simulink model "untitled"  (R2021a)
settings: Solver=FixedStepAuto  StartTime=0.0  StopTime=20  FixedStep=0.1  RelTol=1e-3
undefined symbols (not defined in the file): sigbuilder_block
settings Model: Creator=se108102  LastModifiedBy=se108102

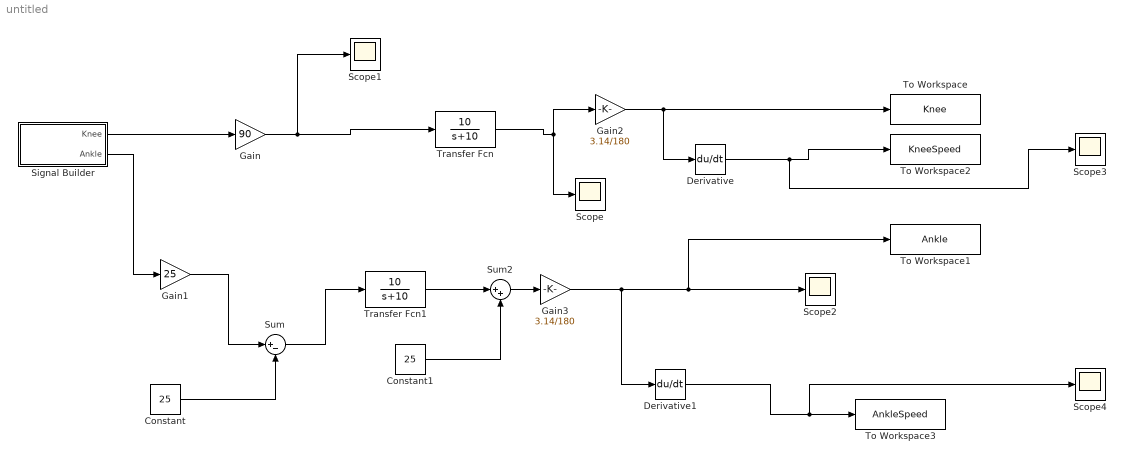
== system untitled ==
  Constant : Constant  Value=25
  Constant1 : Constant  Value=25
  Derivative : Derivative
  Derivative1 : Derivative
  Gain : Gain  Gain=90
  Gain1 : Gain  Gain=25
  Gain2 : Gain  Gain=3.14/180
  Gain3 : Gain  Gain=3.14/180
  Scope{,1..4} (5 alike) : Scope
  Signal Builder : Subsystem  Tag=STV Subsys  LoadFcn=sigbuilder_block('load');  StartFcn=sigbuilder_block('start');  StopFcn=sigbuilder_block('stop');  ClipboardFcn=sigbuilder_block('clipboard');  mask(Sigbuilder block){tuvar=[0:10]}
      mask help: Simulink:masks:SigbuilderBlock_MD
      mask init:
      | if ~strcmp(get_param(bdroot(gcbh),'SimulationStatus'),'stopped') tuvar = sigbuilder_block('maskInit'); end
      settings: CopyFcn=sigbuilder_block('copy');  DeleteFcn=sigbuilder_block('delete');  ModelCloseFcn=sigbuilder_block('modelClose');  PreSaveFcn=sigbuilder_block('preSave');  PauseFcn=sigbuilder_block('pause');  ContinueFcn=sigbuilder_block('continue');  NameChangeFcn=sigbuilder_block('namechange');  OpenFcn=sigbuilder_block('open',[261.75 204.75 602.25 475.5 ]);  CloseFcn=sigbuilder_block('close');
      mask Display: plot(0, 0, 100, 100,[2, 2, 32, 32, 2], [68, 8, 8, 68, 68],[32, 2], [38, 38], [32, 19, 2],[53, 60, 44], [32, 17, 17, 2],[16, 16, 31, 31]);txt = getActiveGroup(gcbh);text(2, 100, txt,'verticalAlignment', 'top');
  Sum : Sum  Inputs=|+-
  Sum2 : Sum  Inputs=|++
  To Workspace : ToWorkspace  VariableName=Knee  SampleTime=-1
  To Workspace1 : ToWorkspace  VariableName=Ankle  SampleTime=-1
  To Workspace2 : ToWorkspace  VariableName=KneeSpeed  SampleTime=-1
  To Workspace3 : ToWorkspace  VariableName=AnkleSpeed  SampleTime=-1
  Transfer Fcn : TransferFcn  Numerator=[10]  Denominator=[1 10]
  Transfer Fcn1 : TransferFcn  Numerator=[10]  Denominator=[1 10]  AbsoluteTolerance=Auto
  wires:
  Signal Builder/1(Knee) -> Gain/1
  Gain/1 -> Transfer Fcn/1, Scope1/1
  Transfer Fcn/1 -> Gain2/1, Scope/1
  Constant/1 -> Sum/2
  Gain1/1 -> Sum/1
  Sum/1 -> Transfer Fcn1/1
  Constant1/1 -> Sum2/2
  Transfer Fcn1/1 -> Sum2/1
  Sum2/1 -> Gain3/1
  Derivative/1 -> Scope3/1, To Workspace2/1
  Derivative1/1 -> Scope4/1, To Workspace3/1
  Gain2/1 -> Derivative/1, To Workspace/1
  Gain3/1 -> Derivative1/1, To Workspace1/1, Scope2/1
  Signal Builder/2(Ankle) -> Gain1/1

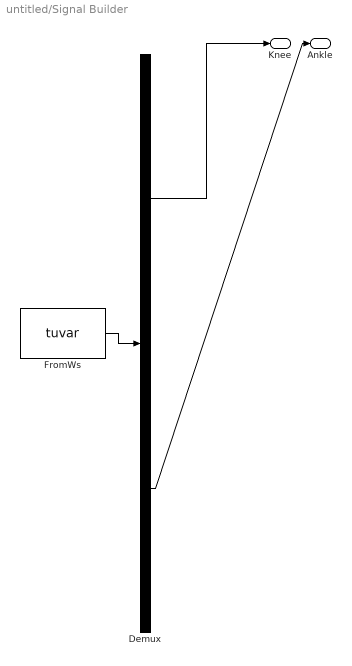
== system untitled/Signal Builder ==
  Demux : Demux  Tag=STV Demux  Outputs=2
      settings: DisplayOption=none
  FromWs : FromWorkspace  Tag=STV FromWs  VariableName=tuvar
      SigBuilderData=|
      | common.afterFinalStr = 'Extrapolate'
      | common.sampleTime = 0
      | dataSet.timeRange = [0 20]
      | dataSet.name = 'Group 1'
      | sbobj.Groups.Name = 'Group 1'
      | sbobj.Groups.Signals(1).Name = 'Knee'
      | sbobj.Groups.Signals(1).XData = [0 2 20]
      | sbobj.Groups.Signals(1).YData = [0 0 1]
      | sbobj.Groups.Signals(2).Name = 'Ankle'
      | sbobj.Groups.Signals(2).XData = [0 2 20]
      | sbobj.Groups.Signals(2).YData = [1 1 0]
      | sbobj.Groups.TimeRange = [0 20]
  Knee : Outport  Tag=STV Outport
  Ankle : Outport  Tag=STV Outport  Port=2
  wires:
  FromWs/1 -> Demux/1
  Demux/1 -> Knee/1
  Demux/2 -> Ankle/1
